simulink model "Exercise_28"  (R2023a)
settings: Solver=VariableStepAuto  StartTime=0.0  StopTime=10  RelTol=1e-3
settings Model: Creator=Admin  LastModifiedBy=Admin

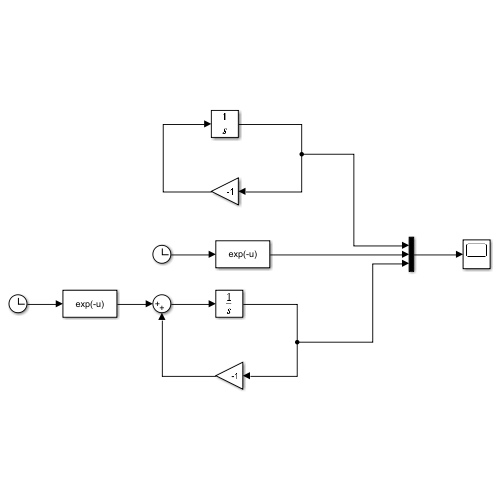
[thumbnail: Simulink's stored preview of the top-level diagram]
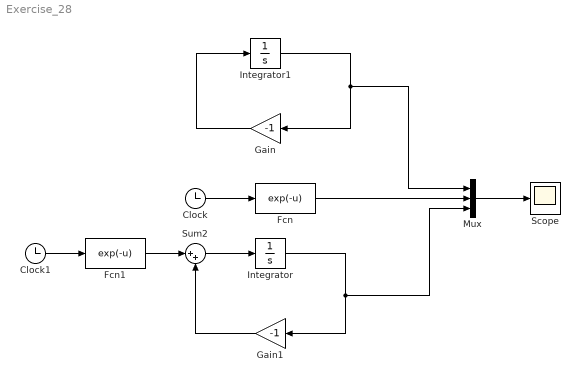
== system Exercise_28 ==
  Clock : Clock
  Clock1 : Clock
  Fcn : Fcn  Expr=exp(-u)
  Fcn1 : Fcn  Expr=exp(-u)
  Gain : Gain  Gain=-1
  Gain1 : Gain  Gain=-1
  Integrator : Integrator  InitialCondition=1
  Integrator1 : Integrator  InitialCondition=1
  Mux : Mux  Inputs=3
  Scope : Scope
  Sum2 : Sum  Inputs=|++
  wires:
  Integrator1/1 -> Gain/1, Mux/1
  Clock/1 -> Fcn/1
  Mux/1 -> Scope/1
  Fcn/1 -> Mux/2
  Integrator/1 -> Gain1/1, Mux/3
  Clock1/1 -> Fcn1/1
  Fcn1/1 -> Sum2/1
  Gain1/1 -> Sum2/2
  Sum2/1 -> Integrator/1
  Gain/1 -> Integrator1/1
